simulink model "magneticField"  (R2023b)
settings: Solver=VariableStepAuto  StartTime=0.0  StopTime=10.0  RelTol=1e-3
settings Model: Creator=kristopherriordan  LastModifiedBy=kristopherriordan

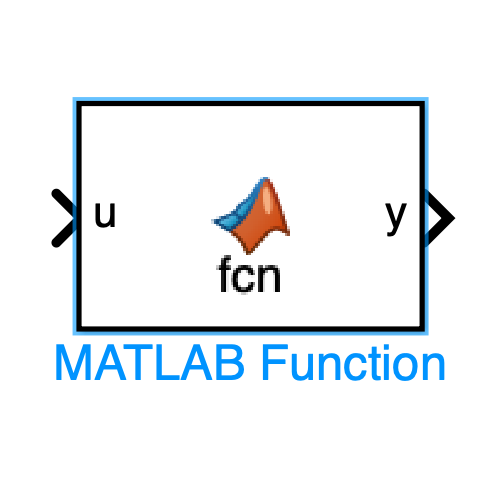
[thumbnail: Simulink's stored preview of the top-level diagram]
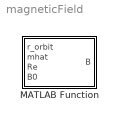
== system magneticField ==
  MATLAB Function : MATLAB Function  TreatAsAtomicUnit=on

== matlab function magneticField/MATLAB Function ==
  data: r_orbit input; B output; mhat input; Re input; B0 input
function B = dipoleMoment(r_orbit, mhat, Re, B0)

R = norm(r_orbit);
Rhat = r_orbit./R;

B = -(Re/R)^3 .* B0 .* (3*(dot(mhat, Rhat).*Rhat) - mhat)


y = u;
